simulink model "LedArray"  (R2015a)
settings: Solver=ode45  StartTime=0.0  StopTime=10.0  RelTol=1e-3
settings Model: Creator=kkhoo  LastModifiedBy=kkhoo

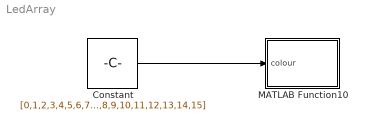
== system LedArray ==
  Constant : Constant  Value=[0,1,2,3,4,5,6,7,8,9,10,11,12,13,14,15]
  MATLAB Function10 : MATLAB Function  LoadFcn=|  TreatAsAtomicUnit=on  mask(IR Send){}
      | set_param(gcs, 'CustomSource', strjoin(unique([strsplit(get_param(gcs, 'CustomSource')) ...
      |  'src/engduino_wrappers.cpp' 'src/Engduino.h'])));
      mask help: Sends one byte at a time using the infrared transmitter.
  wires:
  Constant/1 -> MATLAB Function10/1(colour)

== matlab function LedArray/MATLAB Function10 ==
  data: colour input uint8
function rgb_leds_all_wrapper(colour)

if strcmp(coder.target, 'rtw')
    coder.ceval('ir_send_wrapper', colour);
end
